simulink model "aerosonde_trim"  (Simulink 4.0)
settings: Solver=ode4  SolverMode=SingleTasking  StartTime=0.0  StopTime=TrimParam.FinalTime  FixedStep=TrimParam.SampleTime  RelTol=1e-3
undefined symbols (not defined in the file or in its folder): b, J, TrimParam
libraries: aerosimlib x27, simulink3 x7
settings Model: LastModifiedBy=mariusn  SaveTime=off  SaveOutput=off  LimitDataPoints=off  UnconnectedInputMsg=none  UnconnectedOutputMsg=none  UnconnectedLineMsg=none  BooleanDataType=on

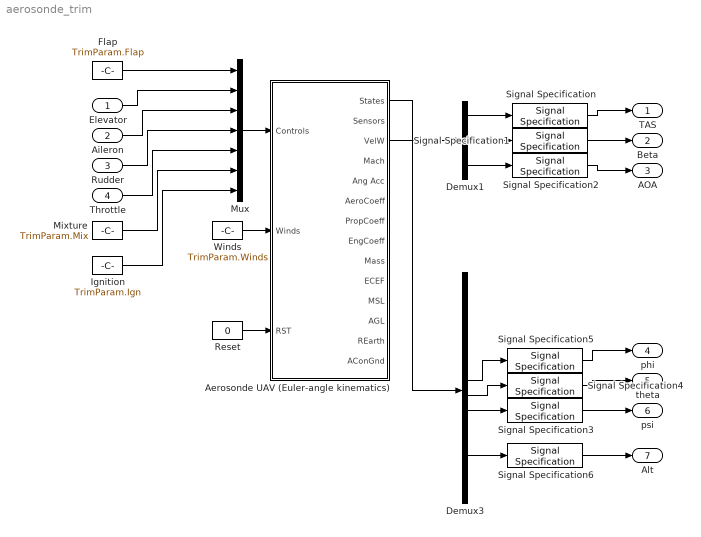
== system aerosonde_trim ==
  Elevator : Inport  Port=1  PortDimensions=-1  SampleTime=-1  DataType=auto
      settings: SignalType=auto
  Aileron : Inport  Port=2  PortDimensions=-1  SampleTime=-1  DataType=auto
      settings: SignalType=auto
  Rudder : Inport  Port=3  PortDimensions=-1  SampleTime=-1  DataType=auto
      settings: SignalType=auto
  Throttle : Inport  Port=4  PortDimensions=-1  SampleTime=-1  DataType=auto
      settings: SignalType=auto
  Aerosonde UAV (Euler-angle kinematics) : Subsystem  SimViewingDevice=off  mask(6-DOF Aircraft Model){aircraftcfg='aerosondecfg.mat', VelocitiesIni=TrimParam.VelocitiesIni, RatesIni=TrimParam.RatesIni, EulerIni=TrimParam.AttitudeIni, PositionIni=TrimParam.PositionIni, FuelIni=TrimParam.FuelIni, OmegaIni=TrimParam.EngineSpeedIni, GndAlt=0, wmmfile='C:\Program Files\AeroSim\wmm.cof', dmy=[08 01 2004], tsamp=TrimParam.SampleTime}
      mask prompts: aircraftcfg "Aircraft configuration file:"; VelocitiesIni "Initial velocities:"; RatesIni "Initial angular rates:"; EulerIni "Initial attitude:"; PositionIni "Initial position:"; FuelIni "Initial fuel mass:"; OmegaIni "Initial engine speed:"; GndAlt "Ground altitude:"; wmmfile "WMM coefficient file:"; dmy "Simulation date:"; tsamp "Sample time:"
      mask help: Nonlinear 6-DOF aircraft model with equations of motion in body frame.
      mask init:
      | load(aircraftcfg);
      settings: Permissions=ReadWrite  RTWFcnNameOpts=Auto  RTWFileNameOpts=Auto
      mask Help:
      | The block implements the 6-DOF nonlinear aircraft model using AeroSim blocks. Velocities are computed in body frame.
      | <P><B>Inputs:</B>
      | <LI>Controls = the 7x1 vector of aircraft controls [flap elevator aileron rudder throttle mixture ignition]. Aerodynamic controls are in radians, throttle is from 0 to 1, mixture is fraction air/fuel flow, ignition is 0 (engine off) or 1 (engine on).</LI>
      | <LI>Winds = the 3x1 vector of background wind speed components in navigation frame [North East Down]</LI>
      | <LI>RST = the integrator reset flag (0 or 1, all integrators on rising edge)
      | </P>
      | <P><B>Outputs:</B>
      | <LI>States = the 15x1 aircraft state vector [Velocities, Angular rates, Quaternions, Position, Fuel mass, Engine speed].</LI>
      | <LI>Sensors = the 18x1 vector of sensor outputs [GPS Position, GPS Groundspeed, Accelerometers, Gyros, Air data, Magnetometer].</LI>
      | <LI>VelW = the 3x1 vector of aircraft velocity in wind axes [Airspeed, sideslip, angle of attack]</LI>
      | <LI>Mach = the Mach number</LI>
      | <LI>Ang Acc = the 3x1 vector of angular accelerations
      | <LI>Euler = the 3x1 vector of Euler angles (roll, pitch, yaw)</LI>
      | <LI>AeroCoeff = the 6x1 vector of aerodynamic coefficients [CD CY CL Cl Cm Cn]</LI>
      | <LI>PropCoeff = the 3x1 vector of propeller coefficients [J CT CP]</LI>
      | <LI>EngCoeff = the 5x1 vector of engine coefficients [MAP Airflow Fuelflow BSFC Power]</LI>
      | <LI>Mass = the current aircraft mass</LI>
      | <LI>ECEF = 3x1 vector of position of the aircraft in the Earth-centered, Earth-fixed frame</LI>
      | <LI>MSL = the aircraft altitude above mean-sea-level</LI>
      | <LI>AGL = the aircraft altitude above terrain</LI>
      | <LI>REarth = the Earth equivalent radius at current location
      | <LI>AConGnd = the aircraft-on-ground flag (0 if aircraft above ground, 1 if aircraft on the ground)</LI>
      | </P>
      | <P><B>Parameters:</B>
      | <LI>Aircraft configuration file = the MAT-file with aircraft data</LI>
      | <LI>Initial velocities = the 3x1 vector of initial aircraft velocities in body axes [u v w]</LI>
      | <LI>Initial angular rates = the 3x1 vector of initial angular rates [p q r]</LI>
      | <LI>Initial attitude = the 4x1 vector of initial quaternions [e0 ex ey ez]</LI>
      | <LI>Initial position = the 3x1 vector of initial aircraft location [Lat Lon Alt]</LI>
      | <LI>Initial fuel mass = the initial quantity of fuel on-board the aircraft</LI>
      | <LI>Initial engine speed = the initial engine rotation speed</LI>
      | <LI>Ground altitude = the ground altitude at aircraft location</LI>
      | <LI>WMM coefficient file = the path to the magnetic model coefficient file</LI>
      | <LI>Simulation date = the date to be used for the magnetic model [day month year]</LI>
      | <LI>Sample time = the aircraft model sample time.</LI>
      | </P>
  Demux1 : Demux  Outputs=3  BusSelectionMode=off
  Demux3 : Demux  Outputs=14  BusSelectionMode=off
  Flap : Constant  Value=TrimParam.Flap
  Ignition : Constant  Value=TrimParam.Ign
  Mixture : Constant  Value=TrimParam.Mix
  Mux : Mux  Inputs=7
  Reset : Constant  Value=0
  Signal Specification{,1..6} (7 alike) : simulink3/Signals & Systems/Signal Specification  D=1  Ts=-1  DataType=double
  Winds : Constant  Value=TrimParam.Winds
  TAS : Outport  Port=1
  Beta : Outport  Port=2
  AOA : Outport  Port=3
  phi : Outport  Port=4
  theta : Outport  Port=5
  psi : Outport  Port=6
  Alt : Outport  Port=7
  wires:
  Mux/1 -> Aerosonde UAV (Euler-angle kinematics)/1(Controls)
  Flap/1 -> Mux/1
  Elevator/1 -> Mux/2
  Aileron/1 -> Mux/3
  Rudder/1 -> Mux/4
  Throttle/1 -> Mux/5
  Mixture/1 -> Mux/6
  Ignition/1 -> Mux/7
  Winds/1 -> Aerosonde UAV (Euler-angle kinematics)/2(Winds)
  Reset/1 -> Aerosonde UAV (Euler-angle kinematics)/3(RST)
  Aerosonde UAV (Euler-angle kinematics)/3(VelW) -> Demux1/1
  Demux1/2 -> Signal Specification1/1
  Demux1/1 -> Signal Specification/1
  Demux1/3 -> Signal Specification2/1
  Aerosonde UAV (Euler-angle kinematics)/1(States) -> Demux3/1
  Demux3/12 -> Signal Specification6/1
  Demux3/7 -> Signal Specification5/1
  Demux3/8 -> Signal Specification4/1
  Demux3/9 -> Signal Specification3/1
  Signal Specification/1 -> TAS/1
  Signal Specification1/1 -> Beta/1
  Signal Specification2/1 -> AOA/1
  Signal Specification5/1 -> phi/1
  Signal Specification4/1 -> theta/1
  Signal Specification3/1 -> psi/1
  Signal Specification6/1 -> Alt/1

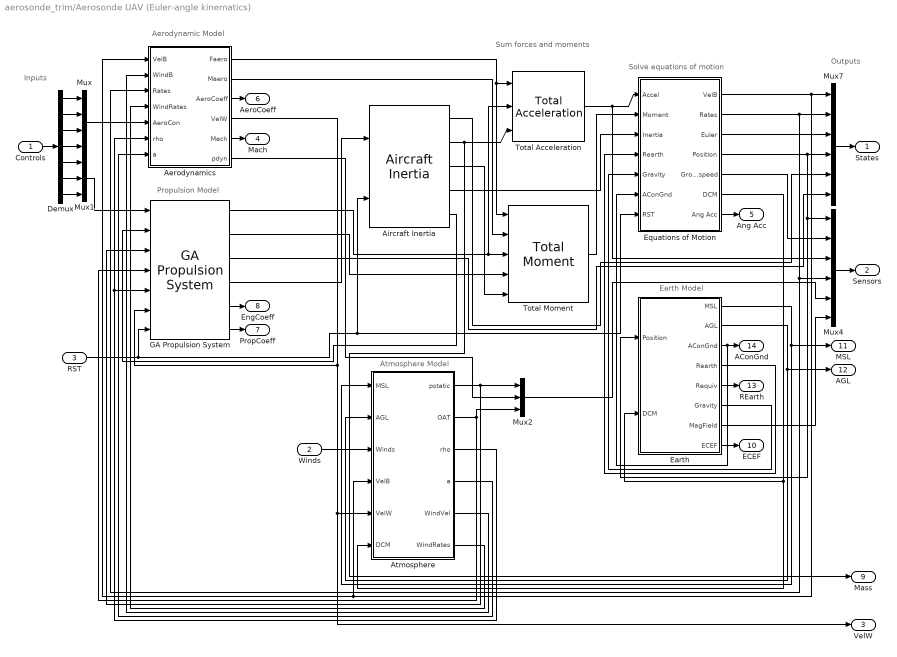
== system aerosonde_trim/Aerosonde UAV (Euler-angle kinematics) ==
  note: Solve equations of motion
  note: Inputs
  note: Outputs
  note: Aerodynamic Model
  note: Earth Model
  note: Sum forces and moments
  note: Atmosphere Model
  note: Propulsion Model
  Controls : Inport  Port=1  PortDimensions=-1  SampleTime=-1  DataType=auto
      settings: SignalType=auto
  Winds : Inport  Port=2  PortDimensions=-1  SampleTime=-1  DataType=auto
      settings: SignalType=auto
  RST : Inport  Port=3  PortDimensions=-1  SampleTime=-1  DataType=auto
      settings: SignalType=auto
  Aerodynamics : Subsystem  SimViewingDevice=off
      settings: Permissions=ReadWrite  RTWFcnNameOpts=Auto  RTWFileNameOpts=Auto
  Aircraft Inertia : aerosimlib/Inertia/Aircraft Inertia  FuelIni=FuelIni  Mempty=mempty  Mgross=mgross  CGempty=CGempty  CGgross=CGgross  Jempty=Jempty  Jgross=Jgross
  Atmosphere : Subsystem  SimViewingDevice=off
      settings: Permissions=ReadWrite  RTWFcnNameOpts=Auto  RTWFileNameOpts=Auto
  Demux : Demux  Outputs=7  BusSelectionMode=off
  Earth : Subsystem  SimViewingDevice=off
      settings: Permissions=ReadWrite  RTWFcnNameOpts=Auto  RTWFileNameOpts=Auto
  Equations of Motion : Subsystem  SimViewingDevice=off
      settings: Permissions=ReadWrite  RTWFcnNameOpts=Auto  RTWFileNameOpts=Auto
  GA Propulsion System : aerosimlib/Propulsion/GA Propulsion System  OmegaIni=OmegaIni  RPM=RPM  MAP=MAP  FuelFlow=FuelFlow  Power=Power  Jeng=Jeng  J=J  CT=CT  CP=CP  Rprop=Rprop  Jprop=Jprop  TSL=TSL
  Mux : Mux  Inputs=4
  Mux1 : Mux  Inputs=3
  Mux2 : Mux  Inputs=3
  Mux4 : Mux  Inputs=6
  Mux7 : Mux  Inputs=6
  Total Acceleration : aerosimlib/Equations of Motion/Total Acceleration
  Total Moment : aerosimlib/Equations of Motion/Total Moment  raero=rAC  rprop=rHub
  States : Outport  Port=1
  Sensors : Outport  Port=2
  VelW : Outport  Port=3
  Mach : Outport  Port=4
  Ang Acc : Outport  Port=5
  AeroCoeff : Outport  Port=6
  PropCoeff : Outport  Port=7
  EngCoeff : Outport  Port=8
  Mass : Outport  Port=9
  ECEF : Outport  Port=10
  MSL : Outport  Port=11
  AGL : Outport  Port=12
  REarth : Outport  Port=13
  AConGnd : Outport  Port=14
  wires:
  Equations of Motion/7(Ang Acc) -> Ang Acc/1
  RST/1 -> Aircraft Inertia/2, Equations of Motion/7(RST), GA Propulsion System/7
  Aircraft Inertia/5 -> GA Propulsion System/2
  Earth/2(AGL) -> AGL/1, Atmosphere/2(AGL)
  Earth/1(MSL) -> MSL/1, Atmosphere/1(MSL)
  Aerodynamics/4(VelW) -> GA Propulsion System/6, VelW/1, Atmosphere/5(VelW)
  GA Propulsion System/4 -> Aircraft Inertia/1
  GA Propulsion System/3 -> Mux7/6
  Aircraft Inertia/1 -> Mux7/5
  Mux2/1 -> Mux4/5
  Aerodynamics/6(pdyn) -> Mux2/2
  Equations of Motion/6(DCM) -> Earth/2(DCM), Atmosphere/6(DCM)
  GA Propulsion System/2 -> Total Moment/4
  GA Propulsion System/1 -> Total Moment/3, Total Acceleration/2
  Aerodynamics/2(Maero) -> Total Moment/2
  Aerodynamics/1(Faero) -> Total Moment/1, Total Acceleration/1
  Aircraft Inertia/3 -> Total Moment/5
  Total Moment/1 -> Equations of Motion/2(Moment)
  Aircraft Inertia/4 -> Equations of Motion/3(Inertia)
  Aircraft Inertia/2 -> Mass/1, Total Acceleration/3
  Earth/4(Rearth) -> Equations of Motion/4(Rearth)
  Earth/6(Gravity) -> Equations of Motion/5(Gravity)
  Earth/7(MagField) -> Mux4/6
  Total Acceleration/1 -> Mux4/3, Equations of Motion/1(Accel)
  Equations of Motion/5(Groundspeed) -> Mux4/2
  Earth/3(AConGnd) -> Equations of Motion/6(AConGnd), AConGnd/1
  Earth/5(Requiv) -> REarth/1
  GA Propulsion System/6 -> PropCoeff/1
  GA Propulsion System/5 -> EngCoeff/1
  Demux/7 -> Mux1/3
  Demux/6 -> Mux1/2
  Demux/5 -> Mux1/1
  Demux/4 -> Mux/4
  Demux/3 -> Mux/3
  Demux/2 -> Mux/2
  Demux/1 -> Mux/1
  Controls/1 -> Demux/1
  Mux4/1 -> Sensors/1
  Mux7/1 -> States/1
  Mux1/1 -> GA Propulsion System/1
  Equations of Motion/1(VelB) -> Mux7/1, Aerodynamics/1(VelB), Atmosphere/4(VelB)
  Equations of Motion/2(Rates) -> Mux4/4, Aerodynamics/3(Rates), Mux7/2
  Equations of Motion/4(Position) -> Earth/1(Position), Mux4/1, Mux7/4
  Mux/1 -> Aerodynamics/5(AeroCon)
  Equations of Motion/3(Euler) -> Mux7/3
  Aerodynamics/5(Mach) -> Mach/1
  Aerodynamics/3(AeroCoeff) -> AeroCoeff/1
  Earth/8(ECEF) -> ECEF/1
  Atmosphere/1(pstatic) -> Mux2/1, GA Propulsion System/3
  Atmosphere/2(OAT) -> Mux2/3, GA Propulsion System/4
  Atmosphere/3(rho) -> Aerodynamics/6(rho), GA Propulsion System/5
  Atmosphere/4(a) -> Aerodynamics/7(a)
  Atmosphere/5(WindVel) -> Aerodynamics/2(WindB)
  Atmosphere/6(WindRates) -> Aerodynamics/4(WindRates)
  Winds/1 -> Atmosphere/3(Winds)

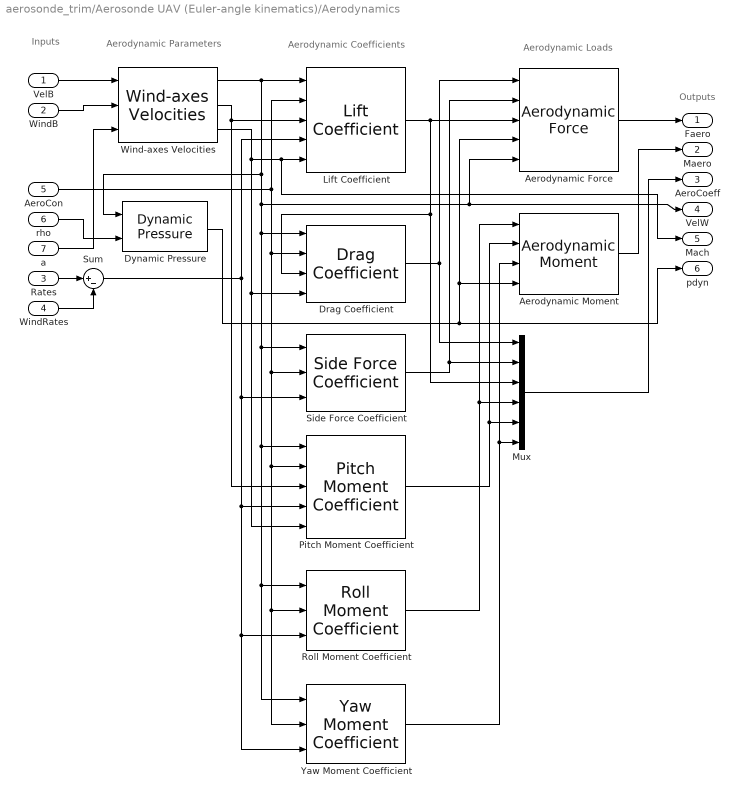
== system aerosonde_trim/Aerosonde UAV (Euler-angle kinematics)/Aerodynamics ==
  note: Inputs
  note: Outputs
  note: Aerodynamic Parameters
  note: Aerodynamic Coefficients
  note: Aerodynamic Loads
  VelB : Inport  Port=1  PortDimensions=[3 1]  SampleTime=-1  DataType=auto
      settings: SignalType=auto
  WindB : Inport  Port=2  PortDimensions=[3 1]  SampleTime=-1  DataType=auto
      settings: SignalType=auto
  Rates : Inport  Port=3  PortDimensions=[3 1]  SampleTime=-1  DataType=auto
      settings: SignalType=auto
  WindRates : Inport  Port=4  PortDimensions=[3 1]  SampleTime=-1  DataType=auto
      settings: SignalType=auto
  AeroCon : Inport  Port=5  PortDimensions=[4 1]  SampleTime=-1  DataType=auto
      settings: SignalType=auto
  rho : Inport  Port=6  PortDimensions=1  SampleTime=-1  DataType=auto
      settings: SignalType=auto
  a : Inport  Port=7  PortDimensions=1  SampleTime=-1  DataType=auto
      settings: SignalType=auto
  Aerodynamic Force : aerosimlib/Aerodynamics/Aerodynamic Force  S=S
  Aerodynamic Moment : aerosimlib/Aerodynamics/Aerodynamic Moment  c=MAC  b=b  S=S
  Drag Coefficient : aerosimlib/Aerodynamics/Drag Coefficient  CL0=CLmind  CD0=CDmin  CDdf=CDdf  CDde=CDde  CDda=CDda  CDdr=CDdr  CDM=CDM  e=osw  b=b  S=S
  Dynamic Pressure : aerosimlib/Aerodynamics/Dynamic Pressure
  Lift Coefficient : aerosimlib/Aerodynamics/Lift Coefficient  CL0=CL0  CLalpha=CLa  CLdf=CLdf  CLde=CLde  CLalphadot=CLalphadot  CLq=CLq  CLM=CLM  c=MAC
  Mux : Mux  Inputs=6
  Pitch Moment Coefficient : aerosimlib/Aerodynamics/Pitch Moment Coefficient  Cm0=Cm0  Cma=Cma  Cmdf=Cmdf  Cmde=Cmde  Cmalphadot=Cmalphadot  Cmq=Cmq  CmM=CmM  c=MAC
  Roll Moment Coefficient : aerosimlib/Aerodynamics/Roll Moment Coefficient  Clbeta=Clbeta  Clda=Clda  Cldr=Cldr  Clp=Clp  Clr=Clr  b=b
  Side Force Coefficient : aerosimlib/Aerodynamics/Side Force Coefficient  CYbeta=CYbeta  CYda=CYda  CYdr=CYdr  CYp=CYp  CYr=CYr  b=b
  Sum : Sum  Inputs=|+-  SaturateOnIntegerOverflow=on
  Wind-axes Velocities : aerosimlib/Aerodynamics/Wind-axes Velocities  Vabnd=VaBnd  betabnd=BetaBnd  alphabnd=AlphaBnd
  Yaw Moment Coefficient : aerosimlib/Aerodynamics/Yaw Moment Coefficient  Cnbeta=Cnbeta  Cnda=Cnda  Cndr=Cndr  Cnp=Cnp  Cnr=Cnr  b=b
  Faero : Outport  Port=1
  Maero : Outport  Port=2
  AeroCoeff : Outport  Port=3
  VelW : Outport  Port=4
  Mach : Outport  Port=5
  pdyn : Outport  Port=6
  wires:
  Sum/1 -> Roll Moment Coefficient/3, Yaw Moment Coefficient/3, Pitch Moment Coefficient/4, Side Force Coefficient/3, Lift Coefficient/4
  WindRates/1 -> Sum/2
  Rates/1 -> Sum/1
  Mux/1 -> AeroCoeff/1
  Aerodynamic Moment/1 -> Maero/1
  Aerodynamic Force/1 -> Faero/1
  Yaw Moment Coefficient/1 -> Mux/6, Aerodynamic Moment/3
  Pitch Moment Coefficient/1 -> Mux/5, Aerodynamic Moment/2
  Roll Moment Coefficient/1 -> Mux/4, Aerodynamic Moment/1
  Dynamic Pressure/1 -> pdyn/1, Aerodynamic Moment/4, Aerodynamic Force/4
  Side Force Coefficient/1 -> Mux/2, Aerodynamic Force/2
  Drag Coefficient/1 -> Mux/1, Aerodynamic Force/1
  Lift Coefficient/1 -> Mux/3, Drag Coefficient/3, Aerodynamic Force/3
  Wind-axes Velocities/3 -> Mach/1, Lift Coefficient/5, Pitch Moment Coefficient/5, Drag Coefficient/4
  Wind-axes Velocities/2 -> Pitch Moment Coefficient/3, Lift Coefficient/3
  AeroCon/1 -> Yaw Moment Coefficient/2, Roll Moment Coefficient/2, Pitch Moment Coefficient/2, Side Force Coefficient/2, Drag Coefficient/2, Lift Coefficient/2
  rho/1 -> Dynamic Pressure/2
  Wind-axes Velocities/1 -> VelW/1, Aerodynamic Force/5, Yaw Moment Coefficient/1, Roll Moment Coefficient/1, Pitch Moment Coefficient/1, Side Force Coefficient/1, Drag Coefficient/1, Dynamic Pressure/1, Lift Coefficient/1
  a/1 -> Wind-axes Velocities/3
  WindB/1 -> Wind-axes Velocities/2
  VelB/1 -> Wind-axes Velocities/1

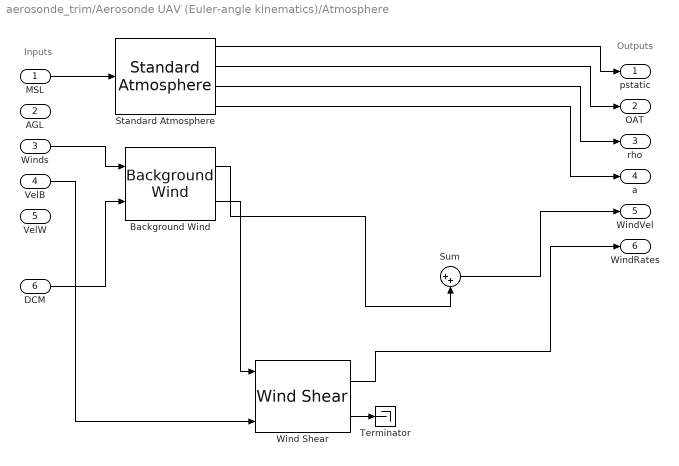
== system aerosonde_trim/Aerosonde UAV (Euler-angle kinematics)/Atmosphere ==
  note: Inputs
  note: Outputs
  MSL : Inport  Port=1  PortDimensions=1  SampleTime=-1  DataType=double
      settings: SignalType=auto
  AGL : Inport  Port=2  PortDimensions=1  SampleTime=-1  DataType=double
      settings: SignalType=auto
  Winds : Inport  Port=3  PortDimensions=[3 1]  SampleTime=-1  DataType=double
      settings: SignalType=auto
  VelB : Inport  Port=4  PortDimensions=[3 1]  SampleTime=-1  DataType=double
      settings: SignalType=auto
  VelW : Inport  Port=5  PortDimensions=[3 1]  SampleTime=-1  DataType=auto
      settings: SignalType=auto
  DCM : Inport  Port=6  PortDimensions=[3 3]  SampleTime=-1  DataType=double
      settings: SignalType=auto
  Background Wind : aerosimlib/Atmosphere/Background Wind
  Standard Atmosphere : aerosimlib/Atmosphere/Standard Atmosphere
  Sum : Sum  Inputs=|++  SaturateOnIntegerOverflow=on
  Terminator : Terminator
  Wind Shear : aerosimlib/Atmosphere/Wind Shear
  pstatic : Outport  Port=1
  OAT : Outport  Port=2
  rho : Outport  Port=3
  a : Outport  Port=4
  WindVel : Outport  Port=5
  WindRates : Outport  Port=6
  wires:
  MSL/1 -> Standard Atmosphere/1
  Winds/1 -> Background Wind/1
  DCM/1 -> Background Wind/2
  Background Wind/1 -> Sum/2
  Background Wind/2 -> Wind Shear/1
  VelB/1 -> Wind Shear/3
  Wind Shear/1 -> WindRates/1
  Standard Atmosphere/1 -> pstatic/1
  Standard Atmosphere/2 -> OAT/1
  Standard Atmosphere/3 -> rho/1
  Standard Atmosphere/4 -> a/1
  Sum/1 -> WindVel/1
  Wind Shear/2 -> Terminator/1

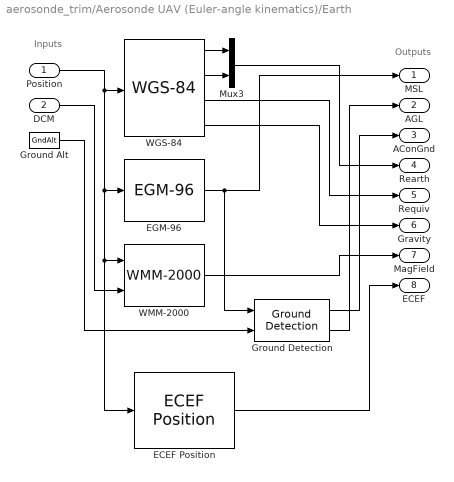
== system aerosonde_trim/Aerosonde UAV (Euler-angle kinematics)/Earth ==
  note: Outputs
  note: Inputs
  Position : Inport  Port=1  PortDimensions=[3 1]  SampleTime=-1  DataType=double
      settings: SignalType=auto
  DCM : Inport  Port=2  PortDimensions=[3 3]  SampleTime=-1  DataType=double
      settings: SignalType=auto
  ECEF Position : aerosimlib/Transformations/ECEF Position
  EGM-96 : aerosimlib/Earth/EGM-96
  Ground Alt : Constant  Value=GndAlt
  Ground Detection : aerosimlib/Earth/Ground Detection
  Mux3 : Mux  Inputs=2
  WGS-84 : aerosimlib/Earth/WGS-84
  WMM-2000 : aerosimlib/Earth/WMM-2000  wmmfile=wmmfile  simdate=dmy
  MSL : Outport  Port=1
  AGL : Outport  Port=2
  AConGnd : Outport  Port=3
  Rearth : Outport  Port=4
  Requiv : Outport  Port=5
  Gravity : Outport  Port=6
  MagField : Outport  Port=7
  ECEF : Outport  Port=8
  wires:
  ECEF Position/1 -> ECEF/1
  WMM-2000/1 -> MagField/1
  WGS-84/4 -> Gravity/1
  WGS-84/3 -> Requiv/1
  Mux3/1 -> Rearth/1
  Ground Detection/1 -> AConGnd/1
  Ground Detection/2 -> AGL/1
  WGS-84/2 -> Mux3/2
  WGS-84/1 -> Mux3/1
  EGM-96/1 -> MSL/1, Ground Detection/1
  Ground Alt/1 -> Ground Detection/2
  DCM/1 -> WMM-2000/2
  Position/1 -> ECEF Position/1, WMM-2000/1, EGM-96/1, WGS-84/1

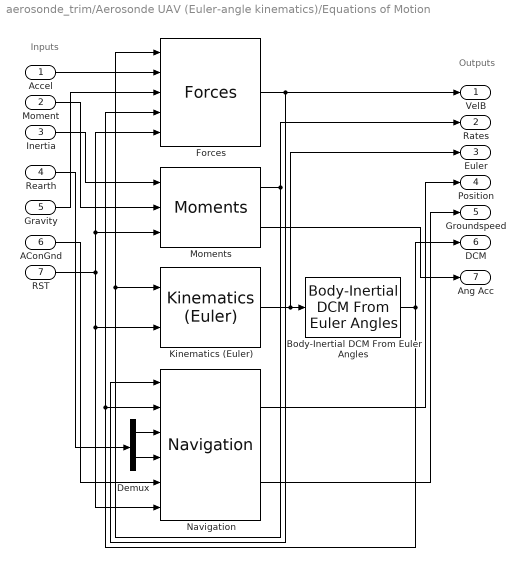
== system aerosonde_trim/Aerosonde UAV (Euler-angle kinematics)/Equations of Motion ==
  note: Inputs
  note: Outputs
  Accel : Inport  Port=1  PortDimensions=[3 1]  SampleTime=-1  DataType=auto
      settings: SignalType=auto
  Moment : Inport  Port=2  PortDimensions=[3 1]  SampleTime=-1  DataType=auto
      settings: SignalType=auto
  Inertia : Inport  Port=3  PortDimensions=[4 1]  SampleTime=-1  DataType=auto
      settings: SignalType=auto
  Rearth : Inport  Port=4  PortDimensions=[2 1]  SampleTime=-1  DataType=auto
      settings: SignalType=auto
  Gravity : Inport  Port=5  PortDimensions=1  SampleTime=-1  DataType=auto
      settings: SignalType=auto
  AConGnd : Inport  Port=6  PortDimensions=1  SampleTime=-1  DataType=auto
      settings: SignalType=auto
  RST : Inport  Port=7  PortDimensions=1  SampleTime=-1  DataType=auto
      settings: SignalType=auto
  Body-Inertial DCM From Euler Angles : aerosimlib/Transformations/Body-Inertial DCM From Euler Angles
  Demux : Demux  Outputs=2  BusSelectionMode=off
  Forces : aerosimlib/Equations of Motion/Body-Frame EOM/Forces  VelocitiesIni=VelocitiesIni
  Kinematics (Euler) : aerosimlib/Equations of Motion/Body-Frame EOM/Kinematics (Euler)  EulerIni=EulerIni
  Moments : aerosimlib/Equations of Motion/Body-Frame EOM/Moments  RatesIni=RatesIni
  Navigation : aerosimlib/Equations of Motion/Body-Frame EOM/Navigation  PositionIni=PositionIni
  VelB : Outport  Port=1
  Rates : Outport  Port=2
  Euler : Outport  Port=3
  Position : Outport  Port=4
  Groundspeed : Outport  Port=5
  DCM : Outport  Port=6
  Ang Acc : Outport  Port=7
  wires:
  Navigation/2 -> Groundspeed/1
  Navigation/1 -> Position/1
  Moments/2 -> Ang Acc/1
  RST/1 -> Navigation/6, Kinematics (Euler)/2, Moments/3, Forces/5
  Moments/1 -> Rates/1, Forces/1, Kinematics (Euler)/1
  Kinematics (Euler)/1 -> Euler/1, Body-Inertial DCM From Euler Angles/1
  Forces/1 -> Navigation/1, VelB/1
  AConGnd/1 -> Navigation/5
  Gravity/1 -> Forces/3
  Inertia/1 -> Moments/1
  Moment/1 -> Moments/2
  Accel/1 -> Forces/2
  Demux/2 -> Navigation/4
  Demux/1 -> Navigation/3
  Rearth/1 -> Demux/1
  Body-Inertial DCM From Euler Angles/1 -> Navigation/2, Forces/4, DCM/1
